simulink model "meam_simulink"  (R2020a)
settings: Solver=FixedStepAuto  StartTime=0.0  StopTime=10.0  FixedStep=0.0001  RelTol=1e-3
undefined symbols (not defined in the file): cnc_comp, ctc_switch, ctrl_at_end, ctrl_space, delta, ea_set_1, ea_set_2, ee_att_1, ee_att_2, f_des, force_ffwd, fp_1, fp_2, frc_comp, grv_comp, ip_1, ip_2, K, Kc, Kd, Kdf, Ki, Kif, Km, Kp, Kpf, orn_at_norm, prdc_frc, q_posIni, q_posIni_1, robot_model_1, robot_model_2, rpt_num_1, rpt_num_2, Sf_diag, spr_comp, switch_val, Sx_diag, tf_1, tf_2, trj_at_end, trj_profile_1, trj_profile_2, trj_space_1, trj_space_2, trj_type_1, trj_type_2
libraries: simulink x2, vrlib x1
(part 4 of 4)

== matlab function meam_simulink/Trajectory Generation1/MATLAB Function1 ==
  data: ip input; fp input; t input; tf input; trj_space input; ea_set input; trj_type input; trj_profile input; rpt_num input; q_pos output; robot_model input; ee_att input; q_vel output; q_acc output; x_pos output; x_vel output; ref input; x_acc output
function [q_pos,q_vel,q_acc,x_pos,x_vel,x_acc] = trj_gen(ip,fp,t,tf,trj_space,ea_set,trj_type,trj_profile,rpt_num,robot_model,ee_att,ref)
    
    if t > tf
        t = tf;
    end

    if trj_space == 0
        
        [r_pos,r_vel,r_acc] = p2pTrj(t,tf,trj_profile);
        
        qi = ip;
        qf = fp;
        
        D = qf - qi;

        q_pos = qi + r_pos*D;
        q_vel = r_vel*D;
        q_acc = r_acc*D;
        
        % forward kinematics
        
        [a_i,alpha_i,d_i,thetaPlus_i] = kinematicParametersOrigin(robot_model);

        [T0_h,~] = forwardGeometry(a_i,alpha_i,d_i,thetaPlus_i+q_pos);

        d_e = getEElength(ee_att);

        Tn_E = [1 0 0 0
                0 1 0 0
                0 0 1 d_e
                0 0 0 1];
            
        T0_E = T0_h(:,:,end)*Tn_E;
    
        t_pos = T0_E(1:3,4);

        J_e = jacobian(a_i,d_i,d_e,q_pos);

        r_posDC = [T0_E(1:3,1);T0_E(1:3,2);T0_E(1:3,3)];

        J_eDot = jacobianDot(a_i,d_i,d_e,q_pos,q_vel);

        x_pos = [t_pos;r_posDC];
        x_vel = J_e*q_vel;
        x_acc = J_eDot*q_vel + J_e*q_acc;

    else
        
        p_ei = ip(1:3);
        r_ei = ip(4:6);
        p_ef = fp(1:3);
        r_ef = fp(4:6);

        Dp = p_ef - p_ei;
        Dr = r_ef - r_ei;
        
        if trj_type ~= 1
            
            [r_pos,r_vel,r_acc] = p2pTrj(t,tf,trj_profile);
            
            t_pos   = p_ei + r_pos*Dp;
            r_posEA = r_ei + r_pos*Dr;

            t_vel   = r_vel*Dp;
            r_velEA = r_vel*Dr;

            t_acc   = r_acc*Dp;
            r_accEA = r_acc*Dr;

        else
            
            period = tf/rpt_num;
            
            Dp = p_ef - p_ei;
            Dr = r_ef - r_ei;
            
            f = (2*pi) / period;
            t_velMax = (Dp*f) / 2.0;
            r_velMax = (Dr*f) / 2.0;
            
            t_pos = p_ei + t_velMax * (1 - cos(f*t)) / f;
            t_vel = t_velMax * sin(f*t);
            t_acc = t_velMax * f * cos(f*t);
            
            r_posEA = r_ei + r_velMax * (1 - cos(f*t)) / f;
            r_velEA = r_velMax * sin(f*t);
            r_accEA = r_velMax * f * cos(f*t);
            
        end
        
        R_e     = getRotMatfromEA(r_posEA,ea_set);

        r_posDC = [R_e(:,1);R_e(:,2);R_e(:,3)];

        E_R     = getE_Rmatrix(r_posEA,ea_set);

        r_velAV = E_R*r_velEA;

        E_RDot  = getE_RDotmatrix(r_posEA,r_velEA,ea_set);
        
        r_accAV = E_RDot*r_velEA+E_R*r_accEA;
        
        x_pos = [t_pos;r_posDC];        
        x_vel = [t_vel;r_velAV];
        x_acc = [t_acc;r_accAV];
        
        % inverse kinematics
        p_e = t_pos;
        
        T0_E = [R_e, p_e;zeros(1,3) 1];

        q_ref = ref(1:6);
        
        [a_i,alpha_i,d_i,thetaPlus_i] = kinematicParametersOrigin(robot_model);

        d_e = getEElength(ee_att);

        q_pos = invGeo(T0_E,a_i,alpha_i,d_i,d_e,thetaPlus_i,q_ref,1);

        J_eInv = inv_jacobian(a_i,d_i,d_e,q_pos);

        q_vel = J_eInv*x_vel;
        
        J_eDot = jacobianDot(a_i,d_i,d_e,q_pos,q_vel);

        q_acc = J_eInv * (x_acc - (J_eDot*q_vel));
    end

    function [r_pos,r_vel,r_acc] = p2pTrj(t,tf,trj_profile)
        
        switch trj_profile
            case 1
                r_pos = t/tf;
                r_vel = 1/tf;
                r_acc = 0;
            case 2
                r_pos = 3*(t/tf)^2 - 2*(t/tf)^3;
                r_vel = 6*(t/tf^2) - 6*(t^2/tf^3);
                r_acc = 6/tf^2 - 12*(t/tf^3);
            case 3
                r_pos = 10*(t/tf)^3 - 15*(t/tf)^4 + 6*(t/tf)^5;
                r_vel = 30*(t^2/tf^3) - 60*(t^3/tf^4) + 30*(t^4/tf^5);
                r_acc = 60*(t/tf^3) - 180*(t^2/tf^4) + 120*(t^3/tf^5);
            case 4
                if t <= tf/2
                    r_pos = 2*(t/tf)^2;
                    r_vel = 4*(t/tf^2);
                    r_acc = 4/tf^2;
                else
                    r_pos = -1 + 4*(t/tf) - 2*(t/tf)^2;
                    r_vel = 4/tf - 4*(t/tf^2);
                    r_acc = -4/tf^2;
                end
            otherwise
                r_pos = 0;
                r_vel = 0;
                r_acc = 0;
        end
        
    end

    function E_R = getE_Rmatrix(r_posEA,eulerSet)
        
        phi = r_posEA(1,1);
        tht = r_posEA(2,1);

        % rotational mapping matrix E_R for euler angles
        E_R = zeros(3,3);
        switch eulerSet
            case 2 % ZYZ
                E_R(1,1) = 0.0;
                E_R(1,2) = -sin(phi);
                E_R(1,3) = cos(phi) * sin(tht);
                E_R(2,1) = 0.0;
                E_R(2,2) = cos(phi);
                E_R(2,3) = sin(phi) * sin(tht);
                E_R(3,1) = 1.0;
                E_R(3,2) = 0.0;
                E_R(3,3) = cos(tht);
            case 3 % ZYX
                E_R(1,1) = 0.0;
                E_R(1,2) = -sin(phi);
                E_R(1,3) = cos(tht) * cos(phi);
                E_R(2,1) = 0.0;
                E_R(2,2) = cos(phi);
                E_R(2,3) = cos(tht) * sin(phi);
                E_R(3,1) = 1.0;
                E_R(3,2) = 0.0;
                E_R(3,3) = -sin(tht);
            case 4 % XYZ
                E_R(1,1) = 1.0;
                E_R(1,2) = 0.0;
                E_R(1,3) = sin(tht);
                E_R(2,1) = 0.0;
                E_R(2,2) = cos(phi);
                E_R(2,3) = -cos(tht) * sin(phi);
                E_R(3,1) = 0.0;
                E_R(3,2) = sin(phi);
                E_R(3,3) = cos(phi) * cos(tht);
            otherwise % ZXZ
                E_R(1,1) = 0.0;
                E_R(1,2) = cos(phi);
                E_R(1,3) = sin(phi) * sin(tht);
                E_R(2,1) = 0.0;
                E_R(2,2) = sin(phi);
                E_R(2,3) = -cos(phi) * sin(tht);
                E_R(3,1) = 1.0;
                E_R(3,2) = 0.0;
                E_R(3,3) = cos(tht);
        end
    end

    function E_RDot = getE_RDotmatrix(r_posEA,r_velEA,eulerSet)
        
        phi = r_posEA(1);
        tht = r_posEA(2);

        phidot = r_velEA(1);
        thtdot = r_velEA(2);

        E_RDot = zeros(3,3);
        switch (eulerSet)
            case 2 % ZYZ
            	E_RDot(1,1) = 0.0;
            	E_RDot(1,2) = -phidot * cos(phi);
            	E_RDot(1,3) = thtdot * cos(phi)*cos(tht) - phidot * sin(phi)*sin(tht);
            	E_RDot(2,1) = 0.0;
            	E_RDot(2,2) = -phidot * sin(phi);
            	E_RDot(2,3) = thtdot * cos(tht)*sin(phi) + phidot * cos(phi)*sin(tht);
            	E_RDot(3,1) = 0.0;
            	E_RDot(3,2) = 0.0;
            	E_RDot(3,3) = -thtdot * sin(tht);
            case 3 % ZYX
            	E_RDot(1,1) = 0.0;
            	E_RDot(1,2) = -phidot * cos(phi);
            	E_RDot(1,3) = -phidot * cos(tht)*sin(phi) - thtdot * cos(phi)*sin(tht);
            	E_RDot(2,1) = 0.0;
            	E_RDot(2,2) = -phidot * sin(phi);
            	E_RDot(2,3) = phidot * cos(phi)*cos(tht) - thtdot * sin(phi)*sin(tht);
            	E_RDot(3,1) = 0.0;
            	E_RDot(3,2) = 0.0;
            	E_RDot(3,3) = -thtdot * cos(tht);
            case 4 %XYZ:
            	E_RDot(1,1) = 0.0;
            	E_RDot(1,2) = 0.0;
            	E_RDot(1,3) = thtdot * cos(tht);
            	E_RDot(2,1) = 0.0;
            	E_RDot(2,2) = -phidot * sin(phi);
            	E_RDot(2,3) = -phidot * cos(phi)*cos(tht) + thtdot * sin(phi)*sin(tht);
            	E_RDot(3,1) = 0.0;
            	E_RDot(3,2) = phidot * cos(phi);
            	E_RDot(3,3) = -phidot * cos(tht)*sin(phi) - thtdot * cos(phi)*sin(tht);
            otherwise % ZXZ
            	E_RDot(1,1) = 0.0;
            	E_RDot(1,2) = -phidot * sin(phi);
            	E_RDot(1,3) = thtdot * cos(tht)*sin(phi) + phidot * cos(phi)*sin(tht);
            	E_RDot(2,1) = 0.0;
            	E_RDot(2,2) = phidot * cos(phi);
            	E_RDot(2,3) = -thtdot * cos(phi)*cos(tht) + phidot * sin(phi)*sin(tht);
            	E_RDot(3,1) = 0.0;
            	E_RDot(3,2) = 0.0;
            	E_RDot(3,3) = -thtdot * sin(tht);
        end
    end

end

== matlab function meam_simulink/Subsystem/End-to-Base Wrench/spatialTrnsE2B ==
  data: x input; f_desE input; f_des output
function f_des = sptTrnsWrnE2B(x,f_desE)
    
    R_mat = [x(4:6) x(7:9) x(10:12)];
    
    X_r = [R_mat zeros(3,3);zeros(3,3) R_mat];
         
    f_des = X_r*f_desE;
        
end

== matlab function meam_simulink/Subsystem/Base-to-End/spatialTrnsB2E1 ==
  data: q input; x input; a output; aB input
function a = sptTrnsAccB2E(q,x,aB)
    
    a = zeros(6,1);
    q_pos = q(1:6);
    q_vel = q(7:12);

    R_mat = [x(4:6) x(7:9) x(10:12)];
    R_dot = getR0_6dotMatrix(q_pos,q_vel);
    
    X_r_inv     = [R_mat' zeros(3,3);zeros(3,3) R_mat'];
    X_r_dot_inv = [R_dot' zeros(3,3);zeros(3,3) R_dot'];
    
    a = X_r_inv*aB + X_r_dot_inv*x(13:18);
    
end

== matlab function meam_simulink/Subsystem/Motion Controller/Inverse Mass Gain ==
  data: Km input; u input size=6; y output size=6
function y = fcn(Km,u)

    sgn = zeros(6,1);
    
    sgn(1) = u(1)/Km(1);
    sgn(2) = u(2)/Km(2);
    sgn(3) = u(3)/Km(3);
    sgn(4) = u(4)/Km(4);
    sgn(5) = u(5)/Km(5);
    sgn(6) = u(6)/Km(6);

y = sgn;

== matlab function meam_simulink/Subsystem/Force Controller/Inverse Mass Gain ==
  data: Km input; u input size=6; y output size=6
function y = fcn(Km,u)

    f = zeros(6,1);
    
    f(1) = u(1)/Km(1);
    f(2) = u(2)/Km(2);
    f(3) = u(3)/Km(3);
    f(4) = u(4)/Km(4);
    f(5) = u(5)/Km(5);
    f(6) = u(6)/Km(6);

y = f;

== matlab function meam_simulink/Subsystem/Motion Controller/Proportional Gain ==
  data: Kp input; u input size=6; y output size=6
function y = fcn(Kp,u)

    sgn = zeros(6,1);
    
    sgn(1) = Kp(1)*u(1);
    sgn(2) = Kp(2)*u(2);
    sgn(3) = Kp(3)*u(3);
    sgn(4) = Kp(4)*u(4);
    sgn(5) = Kp(5)*u(5);
    sgn(6) = Kp(6)*u(6);

y = sgn;

== matlab function meam_simulink/Subsystem/Base-to-End/spatialTrnsB2E2 ==
  data: x input; y output; v input
function y = sptTrnsTwistB2E(x,v)
    
    R_mat = [x(4:6) x(7:9) x(10:12)];
    
    X_r_inv = [R_mat' zeros(3,3);zeros(3,3) R_mat'];
    
    y = X_r_inv*v;
    
end

== matlab function meam_simulink/Subsystem/Base-to-End Wrench/spatialTrnsB2E ==
  data: x input; f_fbk input; f_fbkE output
function f_fbkE = sptTrnsWrnB2E(x,f_fbk)
    
    R_mat = [x(4:6) x(7:9) x(10:12)];
    
    X_r_inv = [R_mat' zeros(3,3);zeros(3,3) R_mat'];
    
    f_fbkE = X_r_inv*f_fbk;
        
end

== matlab function meam_simulink/Subsystem/Compliance/MATLAB Function ==
  data: y output; des input; Kc input; dXf input
function y = fcn(des,Kc,dXf)

    y = des;

    R_mat = [des(16:18) des(19:21) des(22:24)];
    R_new = R_mat*Rot_x(Kc*dXf(2));

    y(16:18) = R_new(1:3,1);
    y(19:21) = R_new(1:3,2);
    y(22:24) = R_new(1:3,3);
    
    function output = Rot_x(input)
        output = [	1	0           0
                    0	cos(input)  -sin(input)
                    0	sin(input)	cos(input)];
    end

%     function output = Rot_z(input)
%         output = [  cos(input)	-sin(input)	0	0
%                     sin(input)	 cos(input)	0	0
%                     0            0          1	0
%                     0            0          0	1 ];
%     end

end

== matlab function meam_simulink/Subsystem/Force Controller/ctrl switch ==
  data: switch_val input; ctrl_at_end input; y output size=1; f_fbk input
function y = fcn(switch_val,ctrl_at_end,f_fbk)

    if ctrl_at_end == 1
        fc_axis = 3;
    else
        fc_axis = 2;
    end
    
    if f_fbk(fc_axis) < switch_val
        y = 0;
    else
        y = 1;
    end
    
end

== matlab function meam_simulink/Environment/MATLAB Function3 ==
  data: x1 input; ee_att_1 input; x2 input size=18; K input; f_e output
function f_e = collisionModel(x1,ee_att_1,x2,K)

    L_srf = [0.64;0.64;0.00];
    
    T0_E_1 = eye(4);
    T0_E_1(1:3,1) = x1(4:6);
    T0_E_1(1:3,2) = x1(7:9);
    T0_E_1(1:3,3) = x1(10:12);
    T0_E_1(1:3,4) = x1(1:3);

    TI_0_1 = eye(4);
    TI_E_1 = TI_0_1*T0_E_1;
    
    TE_I_1 = eye(4);
    TE_I_1(1:3,1:3) = TI_E_1(1:3,1:3)';
    TE_I_1(1:3,4) = -TI_E_1(1:3,1:3)'*TI_E_1(1:3,4);
    
    T0_E_2 = eye(4);
    T0_E_2(1:3,1) = x2(4:6);
    T0_E_2(1:3,2) = x2(7:9);
    T0_E_2(1:3,3) = x2(10:12);
    T0_E_2(1:3,4) = x2(1:3);

    TI_0_2 = [  1,0,0,-0.28
                0,1,0, 2.43
                0,0,1, 0
                0,0,0, 1	];
            
    TI_E_2 = TI_0_2*T0_E_2;
    
    o_e1 = TI_E_1(1:3,4);
    o_e2 = TI_E_2(1:3,4);  
    z_e2 = TI_E_2(1:3,3);
    
    vert_srf_rel = [vertice_2d_gen(zeros(2,1),L_srf(1:2)),ones(4,1)]*TI_E_2'*TE_I_1';

    Mxy = [0,0];
    Axy = [vert_srf_rel(1,1),vert_srf_rel(1,2)];
    Bxy = [vert_srf_rel(2,1),vert_srf_rel(2,2)];
    Cxy = [vert_srf_rel(3,1),vert_srf_rel(3,2)];
    Dxy = [vert_srf_rel(4,1),vert_srf_rel(4,2)];

    coll_xy = pointInTriangle(Axy,Bxy,Cxy,Mxy) || pointInTriangle(Axy,Cxy,Dxy,Mxy);

    D = dot(z_e2,o_e2);

    d = (z_e2(1)*o_e1(1)+z_e2(2)*o_e1(2)+z_e2(3)*o_e1(3)-D)/sqrt(z_e2(1)^2+z_e2(2)^2+z_e2(3)^2);
    
    if ee_att_1 == 3
        if d < 0.0219
            K = 5014;
        end
    end
    
    coll_z = d < 0;
    
    if coll_xy && coll_z
        F = -K*abs(d)*z_e2;    
        f_e = [F(1);F(2);F(3);0;0;0];
    else
        f_e = zeros(6,1);
    end
    
    % floor
    if (o_e1(3) < -0.6)
        f_e(3) = K*(o_e1(3)-0.6);
    end
    
    function vert = vertice_2d_gen(O,L)

        vert = [O(1)-L(1)/2 O(2)-L(2)/2 0; ...
                O(1)-L(1)/2 O(2)+L(2)/2 0; ...
                O(1)+L(1)/2 O(2)+L(2)/2 0; ...
                O(1)+L(1)/2 O(2)-L(2)/2 0];

    end

    function out = pointInTriangle(P1,P2,P3,P)

        denom = ((P2(2) - P3(2))*(P1(1) - P3(1)) + (P3(1) - P2(1))*(P1(2) - P3(2)));

        a = ((P2(2) - P3(2))*(P(1) - P3(1)) + (P3(1) - P2(1))*(P(2) - P3(2))) / denom;
        b = ((P3(2) - P1(2))*(P(1) - P3(1)) + (P1(1) - P3(1))*(P(2) - P3(2))) / denom;
        c = 1 - a - b;

        out = 0 <= a && a <= 1 && 0 <= b && b <= 1 && 0 <= c && c <= 1;

    end

end

== matlab function meam_simulink/Subsystem/Motion Controller/Derivative Gain ==
  data: Kd input; u input size=6; y output size=6
function y = fcn(Kd,u)

    sgn = zeros(6,1);
    
    sgn(1) = Kd(1)*u(1);
    sgn(2) = Kd(2)*u(2);
    sgn(3) = Kd(3)*u(3);
    sgn(4) = Kd(4)*u(4);
    sgn(5) = Kd(5)*u(5);
    sgn(6) = Kd(6)*u(6);

y = sgn;

== matlab function meam_simulink/Subsystem/Motion Controller/Integral Gain ==
  data: Ki input; u input size=6; y output size=6
function y = fcn(Ki,u)

    sgn = zeros(6,1);
    
    sgn(1) = Ki(1)*u(1);
    sgn(2) = Ki(2)*u(2);
    sgn(3) = Ki(3)*u(3);
    sgn(4) = Ki(4)*u(4);
    sgn(5) = Ki(5)*u(5);
    sgn(6) = Ki(6)*u(6);

y = sgn;

== matlab function meam_simulink/Subsystem/Comp/Gravitational ==
  data: robot_model input; ee_att input; g input; q input size=6; tau_grv output size=6
function tau_grv = grvNE(robot_model,ee_att,g,q)

    [a_i,alpha_i,d_i,thetaPlus_i] = kinematicParametersOrigin(robot_model);

    d_e = getEElength(ee_att);

    [~,Th_i] = forwardGeometry(a_i,alpha_i,d_i,thetaPlus_i+q);

    Tn_E = [1 0 0 0
            0 1 0 0
            0 0 1 d_e
            0 0 0 1];

    Th_i(:,:,end) = Th_i(:,:,end)*Tn_E;
    
    Rh_i = zeros(3,3,6+1);
    Rh_i(:,:,1:6) = Th_i(1:3,1:3,:);

    %% Inverse Dynamics
    [m_i,ri_i_ci,Ii_i] = staticInertialParameters(robot_model,ee_att);

    rh_h_i = zeros(3,1,6+1); % +1 because of prcNE
    ci_i = zeros(3,1,6);
    for i1 = 1:6
        % origin i-1 to i on frame i-1
        rh_h_i(:,:,i1) = Th_i(1:3,4,i1);
        ci_i(:,:,i1) = m_i(i1) * ri_i_ci(:,:,i1);
    end
    
    p_obj.rh_h_i = rh_h_i;
    p_obj.ri_i_ci = ri_i_ci;
    p_obj.ci_i = ci_i;
    p_obj.Ii_i = Ii_i;
    p_obj.m_i = m_i;
    q_obj.Rh_i = Rh_i;

    tau_grv = prcNE(p_obj,q_obj,zeros(6,1),zeros(6,1),g);
    
end

== matlab function meam_simulink/Subsystem/Dyn Trns/MATLAB Function ==
  data: robot_model input; ee_att input; u input; tau output; q input
function tau = M_hat(robot_model,ee_att,u,q)

    tau = zeros(6,1);
    
    [a_i,alpha_i,d_i,thetaPlus_i] = kinematicParametersOrigin(robot_model);

    d_e = getEElength(ee_att);

    [~,Th_i] = forwardGeometry(a_i,alpha_i,d_i,thetaPlus_i+q);

    Tn_E = [1 0 0 0
            0 1 0 0
            0 0 1 d_e
            0 0 0 1];

    Th_i(:,:,end) = Th_i(:,:,end)*Tn_E;
    
    Rh_i = zeros(3,3,6+1);
    Rh_i(:,:,1:6) = Th_i(1:3,1:3,:);

    [m_i,ri_i_ci,Ii_i] = staticInertialParameters(robot_model,ee_att);

    rh_h_i = zeros(3,1,6+1); % +1 because of prcNE
    ci_i = zeros(3,1,6);
    for j = 1:6
        % origin i-1 to i on frame i-1
        rh_h_i(:,:,j) = Th_i(1:3,4,j);
        ci_i(:,:,j) = m_i(j) * ri_i_ci(:,:,j);
    end
    
    q_obj.Rh_i = Rh_i;
    p_obj.rh_h_i = rh_h_i;
    p_obj.m_i = m_i;
    p_obj.ci_i = ci_i;
    p_obj.Ii_i = Ii_i;

    v_hat = zeros(6,1);
    M_hat = zeros(6,6);
    for j = 1:6
        if j > 1
            v_hat(j-1) = 0;
        end
        v_hat(j) = 1;
        M_hat(j,:) = prcNE(p_obj,q_obj,zeros(6,1),v_hat,zeros(3,1));
    end
    
    tau = M_hat*u;

end
